simulink model "modulador_torque"  (R2023b)
settings: Solver=VariableStepAuto  StartTime=0.0  StopTime=10.0  RelTol=1e-3
settings Model: Creator=rodri  LastModifiedBy=Nahuel

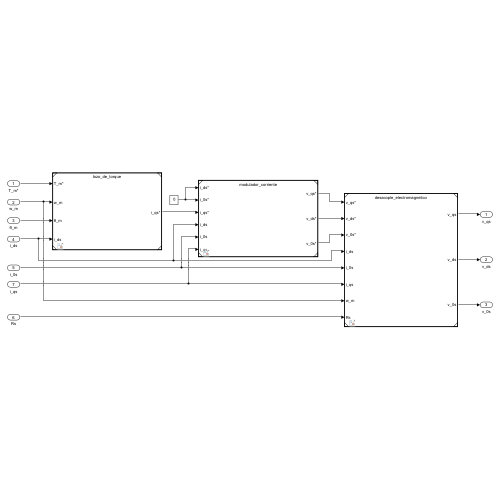
[thumbnail: Simulink's stored preview of the top-level diagram]
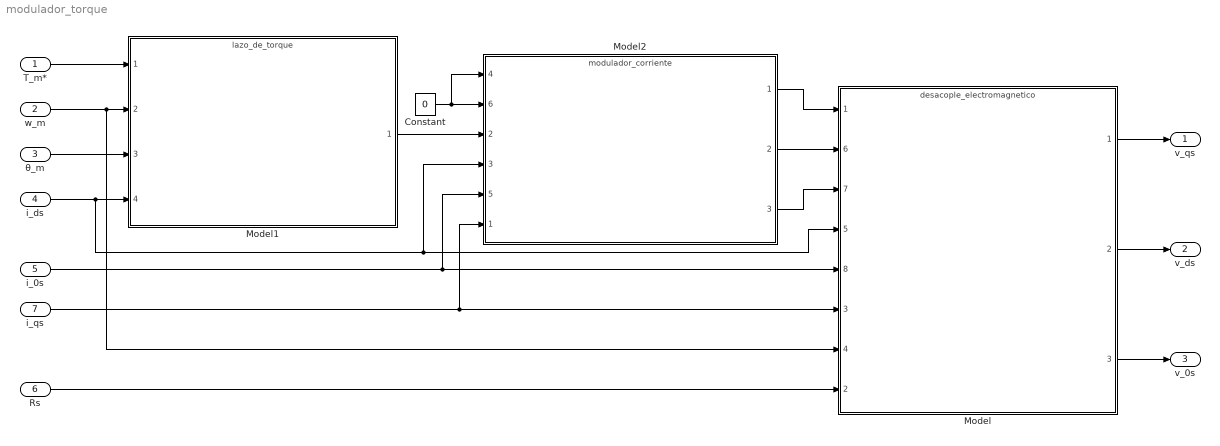
== system modulador_torque ==
  T_m* : Inport
  w_m : Inport  Port=2
  θ_m : Inport  Port=3
  i_ds : Inport  Port=4
  i_0s : Inport  Port=5
  Rs : Inport  Port=6
  i_qs : Inport  Port=7
  Constant : Constant  Value=0
  Model : ModelReference  ModelNameDialog=desacople_electromagnetico.slx  SimulationMode=Normal  ModelReferenceVersion=1.3
      settings: PortSchema="{\"entries\":[{\"content\":{\"sides\":[{\"content\":{\"connectorIds\":[\"In1\",\"In6\",\"In7\",\"In5\",\"In8\",\"In3\",\"In4\",\"In2\"]},\"type\":\"ConnectorPlacement.EquallySpacedRectSide\",\"uuid\":\"173f3cae-e7b6-4614-8530-a40df7e7f488\"},{\"content\":{\"connectorIds\":[\"Out1\",\"Out2\",\"Out3\"],\"side\":\"RIGHT\"},\"type\":\"ConnectorPlacement.EquallySpacedRectSide\",\"uuid\":\"bbd4b6f0-21e5-42a9-8ebb-6dd5e7fed9ab\"},{\"content\":{\"side\":\"TOP\"},\"type\":\"ConnectorPlacement.EquallySpacedRectSide\",\"uuid\":\"98650b14-8bfd-49fa-a2cf-89f0cf3c7bce\"}]},\"type\":\"ConnectorPlacement.EquallySpacedConnector\",\"uuid\":\"07578ec6-06f9-4d1c-b161-452b700d899e\"}],\"packageUris\":[\"http://schema.mathworks.com/mf0/Connector/R2020b\"],\"version\":\"1.0\"}"
  Model1 : ModelReference  ModelNameDialog=lazo_de_torque.slx  SimulationMode=Normal  ModelReferenceVersion=1.2
  Model2 : ModelReference  ModelNameDialog=modulador_corriente.slx  SimulationMode=Normal  ModelReferenceVersion=1.2
      settings: PortSchema="{\"entries\":[{\"content\":{\"sides\":[{\"content\":{\"connectorIds\":[\"In4\",\"In6\",\"In2\",\"In3\",\"In5\",\"In1\"]},\"type\":\"ConnectorPlacement.EquallySpacedRectSide\",\"uuid\":\"aaca9ed2-7705-4604-ba0e-a0ed50227c5d\"},{\"content\":{\"connectorIds\":[\"Out1\",\"Out2\",\"Out3\"],\"side\":\"RIGHT\"},\"type\":\"ConnectorPlacement.EquallySpacedRectSide\",\"uuid\":\"8cc4e0e7-76fd-4770-9995-576aa06169ad\"},{\"content\":{\"side\":\"TOP\"},\"type\":\"ConnectorPlacement.EquallySpacedRectSide\",\"uuid\":\"735fbc83-786f-412b-a6f6-f68ccd2e3496\"}]},\"type\":\"ConnectorPlacement.EquallySpacedConnector\",\"uuid\":\"ed40872b-ad2e-4b2d-a4fe-93f65558232e\"}],\"packageUris\":[\"http://schema.mathworks.com/mf0/Connector/R2020b\"],\"version\":\"1.0\"}"
  v_qs : Outport
  v_ds : Outport  Port=2
  v_0s : Outport  Port=3
  wires:
  Model2/1 -> Model/1
  Model2/2 -> Model/6
  Model2/3 -> Model/7
  T_m*/1 -> Model1/1
  w_m/1 -> Model/4, Model1/2
  θ_m/1 -> Model1/3
  i_ds/1 -> Model/5, Model2/3, Model1/4
  i_0s/1 -> Model/8, Model2/5
  Constant/1 -> Model2/4, Model2/6
  Model1/1 -> Model2/2
  i_qs/1 -> Model2/1, Model/3
  Rs/1 -> Model/2
  Model/1 -> v_qs/1
  Model/2 -> v_ds/1
  Model/3 -> v_0s/1
